simulink model "ADRC_2_order"  (Simulink 7.6)
settings: Solver=ode45  StartTime=0.0  StopTime=500  RelTol=1e-3
settings Model: Creator=Administrator  LastModifiedBy=Administrator
settings DebuggingCC: AlgebraicLoopMsg=none  ArtificialAlgebraicLoopMsg=none  SolverPrmCheckMsg=none  UnknownTsInhSupMsg=none

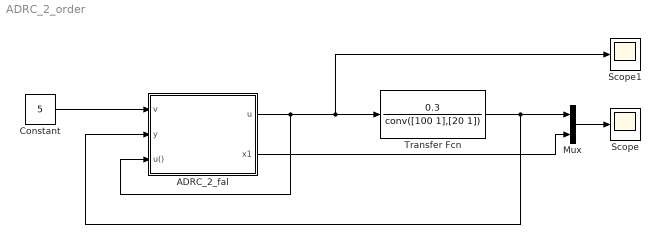
== system ADRC_2_order ==
  ADRC_2_fal : Subsystem  AncestorBlock=ADRC/ADRC/ADRC_2rd/ADRC_2_fal  mask{r=0.0001, h=0.1, B01=20, B02=30, B03=65, D=0.2, b=0.5, k1=5, k2=1, Ds=0.05}
      mask prompts: B01 "B01="; B02 "B02="; B03 "B03="; D "D="; k1 "k1="; k2 "k2="; Ds "Ds="
  Constant : Constant  Value=5
  Mux : Mux  Inputs=2
  Scope : Scope
      settings: TimeRange=500  YMin=-200000  YMax=300000
  Scope1 : Scope
      settings: TimeRange=500  YMin=-1000  YMax=1000
  Transfer Fcn : TransferFcn  Numerator=0.3  Denominator=conv([100 1],[20 1])
  wires:
  Constant/1 -> ADRC_2_fal/1(v)
  Transfer Fcn/1 -> Mux/1, ADRC_2_fal/2(y)
  ADRC_2_fal/1(u) -> ADRC_2_fal/3(u()), Transfer Fcn/1, Scope1/1
  Mux/1 -> Scope/1
  ADRC_2_fal/2(x1) -> Mux/2

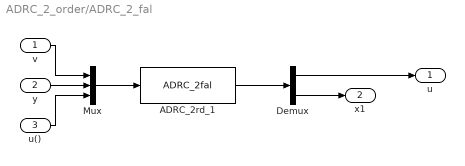
== system ADRC_2_order/ADRC_2_fal ==
  v : Inport
  y : Inport  Port=2
  u() : Inport  Port=3
  ADRC_2rd_1 : S-Function  FunctionName=ADRC_2fal  Parameters=r,h,B01,B02,B03,D,b,k1,k2,Ds  EnableBusSupport=off
  Demux : Demux  Outputs=2
  Mux : Mux  Inputs=3
  u : Outport
  x1 : Outport  Port=2
  wires:
  v/1 -> Mux/1
  y/1 -> Mux/2
  Mux/1 -> ADRC_2rd_1/1
  u()/1 -> Mux/3
  ADRC_2rd_1/1 -> Demux/1
  Demux/1 -> u/1
  Demux/2 -> x1/1
